simulink model "gm_HDLRx_vs"  (R2024a)
settings: Solver=FixedStepDiscrete  StartTime=0.0  StopTime=stopTime  RelTol=1e-3
undefined symbols (not defined in the file or in its folder): channelBitsPerSubcarrier, channelCyclicPrefixLen, channelOFDMSamples, channelScramblerInit, clk, clk_enable, decimatorDelay, decimatorFilter, fPHY, fs, headerBitsPerFec, headerBitsPerSubcarrier, headerCyclicPrefixLen, headerOFDMSamples, headerScramblerInit, lowerbound, N, numDataCarriers, payloadBitsPerFec, payloadScramblerInit, preambleBitsPerSubcarrier, preambleCyclicPrefixLen, preambleFirstPartOFDMSamples, preambleScramblerInit, preambleSecondPartOFDMSamples, QAM, reset_x, upperbound
libraries: hdlsllib x133, hdlmdlgenlib x132, simulink x8, whdlutilities x8, whdlmod x4, dspsrcs4 x2, whdledac x2, commhdlcrc x1, dsphdlfiltering2 x1, dsphdlsigops2 x1, vivadosimlib x1, HDL_ieee_8021513 x1
(part 2 of 4)

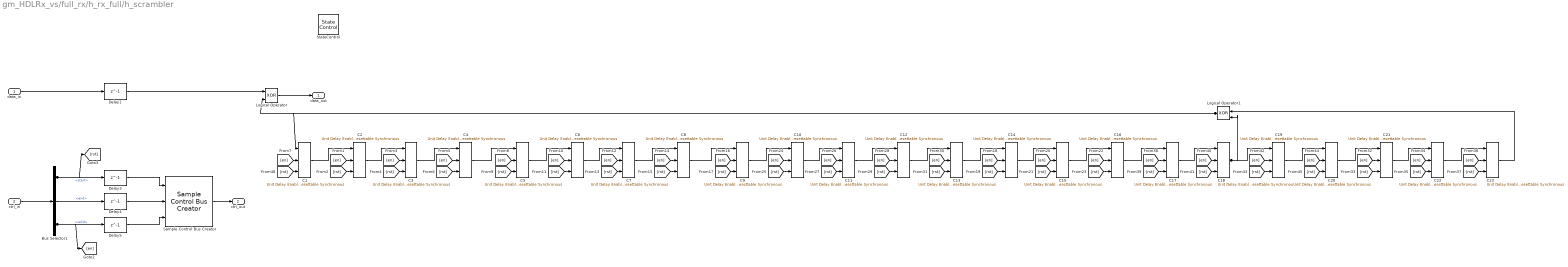
== system gm_HDLRx_vs/full_rx/h_rx_full/h_scrambler ==
  data_in : Inport  OutDataTypeStr=boolean  SampleTime=1e-08
  ctrl_in : Inport  Port=2  SampleTime=1e-08
  Bus Selector1 : BusSelector  OutputSignals=start,end,valid
  C{1,3,5,7,9,11,13,15,17,19,21,23} (12 alike) : hdlsllib/Discrete/Unit Delay Enabled Resettable Synchronous  InitialCondition=0  SampleTime=-1
  C{2,4,6,8,10,12,14,16,18,20,22} (11 alike) : hdlsllib/Discrete/Unit Delay Enabled Resettable Synchronous  InitialCondition=1  SampleTime=-1
  Delay{1,3..5} (4 alike) : Delay  DelayLength=1  InitialCondition=0  UseCircularBuffer=on
  Logical Operator : Logic  Operator=XOR  IconShape=distinctive  AllPortsSameDT=off  OutDataTypeStr=boolean
  Logical Operator1 : Logic  Operator=XOR  IconShape=distinctive  AllPortsSameDT=off  OutDataTypeStr=boolean
  Sample Control Bus Creator : whdlutilities/Sample Control Bus Creator
  StateControl : StateControl  StateControl=Synchronous
  data_out : Outport  SampleTime=1e-08
  ctrl_out : Outport  Port=2  SampleTime=1e-08
  wires:
  Sample Control Bus Creator/1 -> ctrl_out/1
  Logical Operator1/1 -> C1/1, Logical Operator/2
  Logical Operator/1 -> data_out/1
  [rst] -> C5/3
  [en] -> C5/2
  [en] -> C1/2
  [rst] -> C4/3
  [en] -> C4/2
  [rst] -> C1/3
  [rst] -> C20/3
  [en] -> C20/2
  [rst] -> C19/3
  [en] -> C19/2
  [rst] -> C18/3
  [en] -> C18/2
  [rst] -> C3/3
  [rst] -> C17/3
  [en] -> C17/2
  [rst] -> C23/3
  [en] -> C23/2
  [rst] -> C22/3
  [en] -> C22/2
  [rst] -> C21/3
  [en] -> C21/2
  [rst] -> C13/3
  [en] -> C13/2
  [en] -> C3/2
  [rst] -> C12/3
  [en] -> C12/2
  [rst] -> C11/3
  [en] -> C11/2
  [rst] -> C10/3
  [en] -> C10/2
  [rst] -> C16/3
  [en] -> C16/2
  [rst] -> C15/3
  [en] -> C15/2
  [rst] -> C2/3
  [rst] -> C14/3
  [en] -> C14/2
  [rst] -> C9/3
  [en] -> C9/2
  [rst] -> C8/3
  [en] -> C8/2
  [rst] -> C7/3
  [en] -> C7/2
  [rst] -> C6/3
  [en] -> C6/2
  [en] -> C2/2
  Delay5/1 -> Sample Control Bus Creator/3
  Delay4/1 -> Sample Control Bus Creator/2
  Delay3/1 -> Sample Control Bus Creator/1
  Delay1/1 -> Logical Operator/1
  C9/1 -> C10/1
  C8/1 -> C9/1
  C7/1 -> C8/1
  C6/1 -> C7/1
  C5/1 -> C6/1
  C4/1 -> C5/1
  C3/1 -> C4/1
  C23/1 -> Logical Operator1/1
  C22/1 -> C23/1
  C21/1 -> C22/1
  C20/1 -> C21/1
  C2/1 -> C3/1
  C19/1 -> C20/1
  C18/1 -> C19/1, Logical Operator1/2
  C17/1 -> C18/1
  C16/1 -> C17/1
  C15/1 -> C16/1
  C14/1 -> C15/1
  C13/1 -> C14/1
  C12/1 -> C13/1
  C11/1 -> C12/1
  C10/1 -> C11/1
  C1/1 -> C2/1
  Bus Selector1/3 -> Delay5/1, [en]  "<valid>"
  Bus Selector1/2 -> Delay4/1  "<end>"
  Bus Selector1/1 -> Delay3/1, [rst]  "<start>"
  ctrl_in/1 -> Bus Selector1/1
  data_in/1 -> Delay1/1

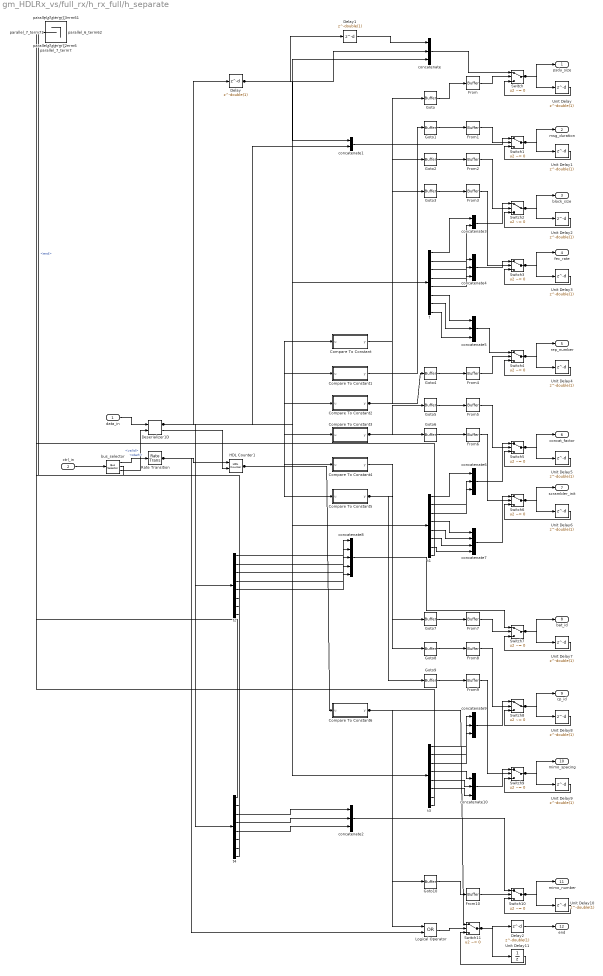
== system gm_HDLRx_vs/full_rx/h_rx_full/h_separate ==
  data_in : Inport  OutDataTypeStr=boolean  SampleTime=1e-08
  ctrl_in : Inport  Port=2  SampleTime=1e-08
  Compare To Constant : Subsystem  mask(Compare To Constant){relop===, const=double(3), OutDataTypeStr=boolean, ZeroCross=on}
      mask prompts: relop "Simulink:masks:Operator_MP"; const "Simulink:masks:ConstantValue_MP"; OutDataTypeStr "Simulink:masks:OutputDataType_MP"; ZeroCross "Simulink:masks:EnableZerocrossingDetection_MP"
      mask help: Simulink:masks:CompareToConstant_MD
      mask init:
      | OutDataTypeStr = 'boolean';
      | ZeroCross = 'on';
      | blkName = 'HDLRx/full_rx/h_rx_full/h_separate/Compare\nTo Constant';
      | const = double(3);
      | const_str = '3';
      | const_val = double(3);
      | relop = '==';
      | setValue = 'boolean';
      | str = '== 3';
      mask TypeOptions relop: == | ~= | < | <= | >= | >
      mask TypeOptions OutDataTypeStr: Simulink:masks:uint8 | Simulink:masks:boolean
      mask Callback ZeroCross: sl('zeroCrossEnable', gcbh);
      mask Display: disp(str)
  Compare To Constant1 : Subsystem  mask(Compare To Constant){relop===, const=double(5), OutDataTypeStr=boolean, ZeroCross=on}
      mask prompts: relop "Simulink:masks:Operator_MP"; const "Simulink:masks:ConstantValue_MP"; OutDataTypeStr "Simulink:masks:OutputDataType_MP"; ZeroCross "Simulink:masks:EnableZerocrossingDetection_MP"
      mask help: Simulink:masks:CompareToConstant_MD
      mask init:
      | OutDataTypeStr = 'boolean';
      | ZeroCross = 'on';
      | blkName = 'HDLRx/full_rx/h_rx_full/h_separate/Compare\nTo Constant1';
      | const = double(5);
      | const_str = '5';
      | const_val = double(5);
      | relop = '==';
      | setValue = 'boolean';
      | str = '== 5';
      mask TypeOptions relop: == | ~= | < | <= | >= | >
      mask TypeOptions OutDataTypeStr: Simulink:masks:uint8 | Simulink:masks:boolean
      mask Callback ZeroCross: sl('zeroCrossEnable', gcbh);
      mask Display: disp(str)
  Compare To Constant2 : Subsystem  mask(Compare To Constant){relop===, const=double(6), OutDataTypeStr=boolean, ZeroCross=on}
      mask prompts: relop "Simulink:masks:Operator_MP"; const "Simulink:masks:ConstantValue_MP"; OutDataTypeStr "Simulink:masks:OutputDataType_MP"; ZeroCross "Simulink:masks:EnableZerocrossingDetection_MP"
      mask help: Simulink:masks:CompareToConstant_MD
      mask init:
      | OutDataTypeStr = 'boolean';
      | ZeroCross = 'on';
      | blkName = 'HDLRx/full_rx/h_rx_full/h_separate/Compare\nTo Constant2';
      | const = double(6);
      | const_str = '6';
      | const_val = double(6);
      | relop = '==';
      | setValue = 'boolean';
      | str = '== 6';
      mask TypeOptions relop: == | ~= | < | <= | >= | >
      mask TypeOptions OutDataTypeStr: Simulink:masks:uint8 | Simulink:masks:boolean
      mask Callback ZeroCross: sl('zeroCrossEnable', gcbh);
      mask Display: disp(str)
  Compare To Constant3 : Subsystem  mask(Compare To Constant){relop===, const=double(7), OutDataTypeStr=boolean, ZeroCross=on}
      mask prompts: relop "Simulink:masks:Operator_MP"; const "Simulink:masks:ConstantValue_MP"; OutDataTypeStr "Simulink:masks:OutputDataType_MP"; ZeroCross "Simulink:masks:EnableZerocrossingDetection_MP"
      mask help: Simulink:masks:CompareToConstant_MD
      mask init:
      | OutDataTypeStr = 'boolean';
      | ZeroCross = 'on';
      | blkName = 'HDLRx/full_rx/h_rx_full/h_separate/Compare\nTo Constant3';
      | const = double(7);
      | const_str = '7';
      | const_val = double(7);
      | relop = '==';
      | setValue = 'boolean';
      | str = '== 7';
      mask TypeOptions relop: == | ~= | < | <= | >= | >
      mask TypeOptions OutDataTypeStr: Simulink:masks:uint8 | Simulink:masks:boolean
      mask Callback ZeroCross: sl('zeroCrossEnable', gcbh);
      mask Display: disp(str)
  Compare To Constant4 : Subsystem  mask(Compare To Constant){relop===, const=double(8), OutDataTypeStr=boolean, ZeroCross=on}
      mask prompts: relop "Simulink:masks:Operator_MP"; const "Simulink:masks:ConstantValue_MP"; OutDataTypeStr "Simulink:masks:OutputDataType_MP"; ZeroCross "Simulink:masks:EnableZerocrossingDetection_MP"
      mask help: Simulink:masks:CompareToConstant_MD
      mask init:
      | OutDataTypeStr = 'boolean';
      | ZeroCross = 'on';
      | blkName = 'HDLRx/full_rx/h_rx_full/h_separate/Compare\nTo Constant4';
      | const = double(8);
      | const_str = '8';
      | const_val = double(8);
      | relop = '==';
      | setValue = 'boolean';
      | str = '== 8';
      mask TypeOptions relop: == | ~= | < | <= | >= | >
      mask TypeOptions OutDataTypeStr: Simulink:masks:uint8 | Simulink:masks:boolean
      mask Callback ZeroCross: sl('zeroCrossEnable', gcbh);
      mask Display: disp(str)
  Compare To Constant5 : Subsystem  mask(Compare To Constant){relop===, const=double(9), OutDataTypeStr=boolean, ZeroCross=on}
      mask prompts: relop "Simulink:masks:Operator_MP"; const "Simulink:masks:ConstantValue_MP"; OutDataTypeStr "Simulink:masks:OutputDataType_MP"; ZeroCross "Simulink:masks:EnableZerocrossingDetection_MP"
      mask help: Simulink:masks:CompareToConstant_MD
      mask init:
      | OutDataTypeStr = 'boolean';
      | ZeroCross = 'on';
      | blkName = 'HDLRx/full_rx/h_rx_full/h_separate/Compare\nTo Constant5';
      | const = double(9);
      | const_str = '9';
      | const_val = double(9);
      | relop = '==';
      | setValue = 'boolean';
      | str = '== 9';
      mask TypeOptions relop: == | ~= | < | <= | >= | >
      mask TypeOptions OutDataTypeStr: Simulink:masks:uint8 | Simulink:masks:boolean
      mask Callback ZeroCross: sl('zeroCrossEnable', gcbh);
      mask Display: disp(str)
  Compare To Constant6 : Subsystem  mask(Compare To Constant){relop===, const=double(13), OutDataTypeStr=boolean, ZeroCross=on}
      mask prompts: relop "Simulink:masks:Operator_MP"; const "Simulink:masks:ConstantValue_MP"; OutDataTypeStr "Simulink:masks:OutputDataType_MP"; ZeroCross "Simulink:masks:EnableZerocrossingDetection_MP"
      mask help: Simulink:masks:CompareToConstant_MD
      mask init:
      | OutDataTypeStr = 'boolean';
      | ZeroCross = 'on';
      | blkName = 'HDLRx/full_rx/h_rx_full/h_separate/Compare\nTo Constant6';
      | const = double(13);
      | const_str = '13';
      | const_val = double(13);
      | relop = '==';
      | setValue = 'boolean';
      | str = '== 13';
      mask TypeOptions relop: == | ~= | < | <= | >= | >
      mask TypeOptions OutDataTypeStr: Simulink:masks:uint8 | Simulink:masks:boolean
      mask Callback ZeroCross: sl('zeroCrossEnable', gcbh);
      mask Display: disp(str)
  Delay : Delay  DelayLength=double(1)  InitialCondition=0  SampleTime=8e-08
  Delay1 : Delay  DelayLength=double(1)  InitialCondition=0  SampleTime=8e-08
  Delay2 : Delay  DelayLength=double(1)  InitialCondition=0  SampleTime=8e-08
  Deserializer1D : hdlsllib/HDL Operations/Deserializer1D  Ratio=8  IdleCycles=0  InitialCondition=0  startIn=off  validIn=on  validOut=on  inputDataDimensions=1  inputSampleTime=1e-08  inputSignalType=real
  From{,1..10} (11 alike) : hdlmdlgenlib/Buffer
  Goto{,1..10} (11 alike) : hdlmdlgenlib/Buffer
  HDL Counter1 : hdlsllib/Sources/HDL Counter  CountType=Free running  CountInit=0  CountStep=1  CountMax=25  CountFromType=Initial value  CountFrom=0  CountResetPort=on  CountLoadPort=off  CountEnbPort=on  CountDirPort=off  CountHitOutputPort=off  CountDataType=Unsigned  CountWordLen=5  CountFracLen=0  CountSampTime=1
  Logical Operator : Logic  Operator=OR  AllPortsSameDT=off  OutDataTypeStr=boolean  SampleTime=8e-08
  Rate Transition : RateTransition  InitialCondition=double(0)  OutPortSampleTimeOpt=Multiple of input port sample time  OutPortSampleTimeMultiple=8
  Switch{,1..10} (11 alike) : Switch  Criteria=u2 ~= 0  Threshold=double(0)  OutDataTypeStr=fixdt(0, 1, 0)  SampleTime=8e-08  SaturateOnIntegerOverflow=off  InputSameDT=off
  Switch11 : Switch  Criteria=u2 ~= 0  Threshold=double(0)  OutDataTypeStr=boolean  SampleTime=8e-08  SaturateOnIntegerOverflow=off  InputSameDT=off
  Unit Delay{,1..10} (11 alike) : Delay  DelayLength=double(1)  InitialCondition=0  SampleTime=8e-08
  Unit Delay11 : UnitDelay  SampleTime=8e-08
  bus_selector : BusSelector  OutputSignals=start,end,valid
  bus_selector_term1 : Terminator
  concatenate{,2,4..6,9..10} (7 alike) : Concatenate  NumInputs=3
  concatenate1 : Concatenate
  concatenate3 : Concatenate
  concatenate7 : Concatenate  NumInputs=4
  concatenate8 : Concatenate  NumInputs=5
  parallel_0_term0 : Terminator
  parallel_1_term1 : Terminator
  parallel_5_term5 : Terminator
  parallel_5_term51 : Terminator
  parallel_6_term6 : Terminator
  parallel_6_term61 : Terminator
  parallel_6_term62 : Terminator
  parallel_7_term{7,71..73} (4 alike) : Terminator
  t{,1..4} (5 alike) : Demux  Outputs=8
  psdu_size : Outport  SampleTime=8e-08
  msg_duration : Outport  Port=2  SampleTime=8e-08
  block_size : Outport  Port=3  SampleTime=8e-08
  fec_rate : Outport  Port=4  SampleTime=8e-08
  rep_number : Outport  Port=5  SampleTime=8e-08
  concat_factor : Outport  Port=6  SampleTime=8e-08
  scrambler_init : Outport  Port=7  SampleTime=8e-08
  bat_id : Outport  Port=8  SampleTime=8e-08
  cp_id : Outport  Port=9  SampleTime=8e-08
  mimo_spacing : Outport  Port=10  SampleTime=8e-08
  mimo_number : Outport  Port=11  SampleTime=8e-08
  end : Outport  Port=12  SampleTime=8e-08
  wires:
  t4/8 -> parallel_7_term7/1
  t4/7 -> parallel_6_term61/1
  t4/6 -> parallel_5_term5/1
  t4/5 -> concatenate2/3
  t4/4 -> concatenate2/2
  t4/3 -> concatenate2/1
  t4/2 -> parallel_1_term1/1
  t4/1 -> parallel_0_term0/1
  t3/8 -> parallel_7_term71/1
  t3/7 -> parallel_6_term62/1
  t3/6 -> concatenate10/3
  t3/5 -> concatenate10/2
  t3/4 -> concatenate10/1
  t3/3 -> concatenate9/3
  t3/2 -> concatenate9/2
  t3/1 -> concatenate9/1
  t2/8 -> parallel_7_term72/1
  t2/7 -> parallel_6_term6/1
  t2/6 -> parallel_5_term51/1
  t2/5 -> concatenate8/5
  t2/4 -> concatenate8/4
  t2/3 -> concatenate8/3
  t2/2 -> concatenate8/2
  t2/1 -> concatenate8/1
  t1/8 -> parallel_7_term73/1
  t1/7 -> concatenate7/4
  t1/6 -> concatenate7/3
  t1/5 -> concatenate7/2
  t1/4 -> concatenate7/1
  t1/3 -> concatenate6/3
  t1/2 -> concatenate6/2
  t1/1 -> concatenate6/1
  t/8 -> concatenate5/3
  t/7 -> concatenate5/2
  t/6 -> concatenate5/1
  t/5 -> concatenate4/3
  t/4 -> concatenate4/2
  t/3 -> concatenate4/1
  t/2 -> concatenate3/2
  t/1 -> concatenate3/1
  Goto9/1 -> From9/1
  Goto8/1 -> From8/1
  Goto7/1 -> From7/1
  Goto6/1 -> From6/1
  Goto5/1 -> From5/1
  Goto4/1 -> From4/1
  Goto3/1 -> From3/1
  Goto2/1 -> From2/1
  Goto10/1 -> From10/1
  Goto1/1 -> From1/1
  Goto/1 -> From/1
  concatenate10/1 -> Switch9/1
  concatenate9/1 -> Switch8/1
  concatenate8/1 -> Switch7/1
  concatenate7/1 -> Switch6/1
  concatenate6/1 -> Switch5/1
  concatenate5/1 -> Switch4/1
  concatenate4/1 -> Switch3/1
  concatenate3/1 -> Switch2/1
  concatenate2/1 -> Switch10/1
  concatenate1/1 -> Switch1/1
  concatenate/1 -> Switch/1
  Unit Delay9/1 -> Switch9/3
  Unit Delay8/1 -> Switch8/3
  Unit Delay7/1 -> Switch7/3
  Unit Delay6/1 -> Switch6/3
  Unit Delay5/1 -> Switch5/3
  Unit Delay4/1 -> Switch4/3
  Unit Delay3/1 -> Switch3/3
  Unit Delay2/1 -> Switch2/3
  Unit Delay11/1 -> Switch11/3
  Unit Delay10/1 -> Switch10/3
  Unit Delay1/1 -> Switch1/3
  Unit Delay/1 -> Switch/3
  Switch9/1 -> mimo_spacing/1, Unit Delay9/1
  Switch8/1 -> cp_id/1, Unit Delay8/1
  Switch7/1 -> bat_id/1, Unit Delay7/1
  Switch6/1 -> scrambler_init/1, Unit Delay6/1
  Switch5/1 -> concat_factor/1, Unit Delay5/1
  Switch4/1 -> rep_number/1, Unit Delay4/1
  Switch3/1 -> fec_rate/1, Unit Delay3/1
  Switch2/1 -> block_size/1, Unit Delay2/1
  Switch11/1 -> Delay2/1, Unit Delay11/1
  Switch10/1 -> mimo_number/1, Unit Delay10/1
  Switch1/1 -> msg_duration/1, Unit Delay1/1
  Switch/1 -> psdu_size/1, Unit Delay/1
  bus_selector/3 -> Deserializer1D/2  "<valid>"
  bus_selector/2 -> bus_selector_term1/1  "<end>"
  bus_selector/1 -> Rate Transition/1  "<start>"
  Rate Transition/1 -> HDL Counter1/1, Logical Operator/2
  Logical Operator/1 -> Switch11/2
  HDL Counter1/1 -> Compare To Constant/1(u), Compare To Constant1/1(u), Compare To Constant2/1(u), Compare To Constant3/1(u), Compare To Constant4/1(u), Compare To Constant5/1(u), Compare To Constant6/1(u)
  From9/1 -> Switch9/2
  From8/1 -> Switch8/2
  From7/1 -> Switch7/2
  From6/1 -> Switch6/2
  From5/1 -> Switch5/2
  From4/1 -> Switch4/2
  From3/1 -> Switch3/2
  From2/1 -> Switch2/2
  From10/1 -> Switch10/2
  From1/1 -> Switch1/2
  From/1 -> Switch/2
  Deserializer1D/2 -> HDL Counter1/2
  Deserializer1D/1 -> Delay/1, t/1, t1/1, t2/1, t3/1, t4/1, concatenate/3, concatenate1/2
  Delay2/1 -> end/1
  Delay1/1 -> concatenate/1
  Delay/1 -> Delay1/1, concatenate/2, concatenate1/1
  Compare To Constant6/1(y) -> Goto10/1, Logical Operator/1, Switch11/1
  Compare To Constant5/1(y) -> Goto8/1, Goto9/1
  Compare To Constant4/1(y) -> Goto7/1
  Compare To Constant3/1(y) -> Goto5/1, Goto6/1
  Compare To Constant2/1(y) -> Goto2/1, Goto3/1, Goto4/1
  Compare To Constant1/1(y) -> Goto1/1
  Compare To Constant/1(y) -> Goto/1
  ctrl_in/1 -> bus_selector/1
  data_in/1 -> Deserializer1D/1

== system gm_HDLRx_vs/full_rx/header_clock_x2/rising_edge_detector ==
  In : Inport  OutDataTypeStr=boolean  SampleTime=1e-08
  Delay2 : Delay  DelayLength=1  InitialCondition=0  UseCircularBuffer=on
  Logical Operator1 : Logic  IconShape=distinctive  AllPortsSameDT=off  OutDataTypeStr=boolean
  Logical Operator2 : Logic  Operator=NOT  IconShape=distinctive  AllPortsSameDT=off  OutDataTypeStr=boolean
  Out : Outport  SampleTime=1e-08
  wires:
  Logical Operator2/1 -> Logical Operator1/2
  Logical Operator1/1 -> Out/1
  Delay2/1 -> Logical Operator2/1
  In/1 -> Delay2/1, Logical Operator1/1

== system gm_HDLRx_vs/full_rx/prepare_payload_data/falling_edge_detector ==
  in : Inport  OutDataTypeStr=boolean  SampleTime=1e-08
  Delay : Delay  DelayLength=1  InitialCondition=0  UseCircularBuffer=on
  Logical Operator : Logic  IconShape=distinctive  AllPortsSameDT=off  OutDataTypeStr=boolean
  Logical Operator1 : Logic  Operator=NOT  IconShape=distinctive  AllPortsSameDT=off  OutDataTypeStr=boolean
  out : Outport  SampleTime=1e-08
  wires:
  Logical Operator1/1 -> Logical Operator/1
  Logical Operator/1 -> out/1
  Delay/1 -> Logical Operator/2
  in/1 -> Delay/1, Logical Operator1/1

== system gm_HDLRx_vs/full_rx/prepare_payload_data/payload_clock_x2 ==
  data_in : Inport  OutDataTypeStr=fixdt(1, 16, 12)  PortDimensions=[4 1]  SampleTime=2e-08
  valid_in : Inport  Port=2  OutDataTypeStr=boolean  PortDimensions=1  SampleTime=2e-08
  Serializer1D : hdlsllib/HDL Operations/Serializer1D  Ratio=2  IdleCycles=0  validIn=on  startOut=off  validOut=on  inputDataDimensions=2  inputSampleTime=2e-08  inputSignalType=real
  concatenate : Concatenate  Mode=Multidimensional array
  data_in_0_term0 : Terminator
  data_in_1_term1 : Terminator
  t : Demux
  data_out : Outport  SampleTime=1e-08
  valid_out : Outport  Port=2  SampleTime=1e-08
  wires:
  t/4 -> concatenate/2
  t/3 -> concatenate/1
  t/2 -> data_in_1_term1/1
  t/1 -> data_in_0_term0/1
  concatenate/1 -> Serializer1D/1
  Serializer1D/2 -> valid_out/1
  Serializer1D/1 -> data_out/1
  valid_in/1 -> Serializer1D/2
  data_in/1 -> t/1

== system gm_HDLRx_vs/full_rx/prepare_payload_data/rising_edge_detector ==
  In : Inport  OutDataTypeStr=boolean  SampleTime=1e-08
  Delay2 : Delay  DelayLength=1  InitialCondition=0  UseCircularBuffer=on
  Logical Operator1 : Logic  IconShape=distinctive  AllPortsSameDT=off  OutDataTypeStr=boolean
  Logical Operator2 : Logic  Operator=NOT  IconShape=distinctive  AllPortsSameDT=off  OutDataTypeStr=boolean
  Out : Outport  SampleTime=1e-08
  wires:
  Logical Operator2/1 -> Logical Operator1/2
  Logical Operator1/1 -> Out/1
  Delay2/1 -> Logical Operator2/1
  In/1 -> Delay2/1, Logical Operator1/1

== system gm_HDLRx_vs/full_rx/rx_demodulator_full/constellation_descrambler ==
  data_in : Inport  OutDataTypeStr=fixdt(1, 24, 12)  SampleTime=2e-08
      settings: SignalType=complex
  valid_in : Inport  Port=2  OutDataTypeStr=boolean  SampleTime=2e-08
  init : Inport  Port=3  OutDataTypeStr=boolean  PortDimensions=[13]  SampleTime=2e-08
  rising_edge_detector : Subsystem
  rotate_-90 : Subsystem
  sync_constellation_scrambler : Subsystem
  data_out : Outport  SampleTime=2e-08
  valid_out : Outport  Port=2  SampleTime=2e-08
  wires:
  sync_constellation_scrambler/2(s2) -> rotate_-90/4(s2_in)
  sync_constellation_scrambler/1(s1) -> rotate_-90/3(s1_in)
  rotate_-90/2(valid_out) -> valid_out/1
  rotate_-90/1(data_out) -> data_out/1
  rising_edge_detector/1(Out) -> sync_constellation_scrambler/1(new_ofdm_symbol)
  init/1 -> sync_constellation_scrambler/2(init)
  valid_in/1 -> sync_constellation_scrambler/3(valid_in), rotate_-90/2(valid_in), rising_edge_detector/1(In)
  data_in/1 -> rotate_-90/1(data_in)

== system gm_HDLRx_vs/full_rx/rx_demodulator_full/decimator ==
  data_in : Inport  OutDataTypeStr=fixdt(1, 16, 12)  SampleTime=1e-08
      settings: SignalType=complex
  valid_in : Inport  Port=2  OutDataTypeStr=boolean  SampleTime=1e-08
  Delay : Delay  InitialCondition=0  UseCircularBuffer=on
  Delay1 : Delay  DelayLength=decimatorDelay/2  InitialCondition=0  UseCircularBuffer=on
  Delay2 : Delay  InitialCondition=0  UseCircularBuffer=on
  Delay3 : Delay  DelayLength=(decimatorDelay-2)*4  InitialCondition=0  UseCircularBuffer=on
  Delay4 : Delay  DelayLength=1  InitialCondition=0  UseCircularBuffer=on
  Delay5 : Delay  DelayLength=1  InitialCondition=0  UseCircularBuffer=on
  FIR Decimator : dsphdlfiltering2/FIR Decimator  Numerator=decimatorFilter.Numerator  FilterStructure=Direct form systolic  DecimationFactor=oversamplingFactor  NumCycles=1  SimulateUsing=Code generation  roundingMode=Floor  overflowMode=off  CoefficientsDataTypeStr=fixdt(1,16)  OutputDataTypeStr=fixdt(1,16,12)  ResetInputPort=on  HDLGlobalReset=off
  Logical Operator : Logic  Operator=OR  IconShape=distinctive  AllPortsSameDT=off  OutDataTypeStr=boolean
  Logical Operator1 : Logic  IconShape=distinctive  AllPortsSameDT=off  OutDataTypeStr=boolean
  Rate Transition : RateTransition  OutPortSampleTimeOpt=Multiple of input port sample time  OutPortSampleTimeMultiple=oversamplingFactor
  Rate Transition1 : RateTransition  OutPortSampleTimeOpt=Multiple of input port sample time  OutPortSampleTimeMultiple=oversamplingFactor
  rising_edge_detector : Subsystem
  data_out : Outport  SampleTime=2e-08
  valid_out : Outport  Port=2  SampleTime=2e-08
  wires:
  rising_edge_detector/1(Out) -> FIR Decimator/3
  Rate Transition1/1 -> data_out/1
  Rate Transition/1 -> Delay1/1, Logical Operator1/1
  Logical Operator1/1 -> valid_out/1
  Logical Operator/1 -> FIR Decimator/2
  FIR Decimator/2 -> Rate Transition/1
  FIR Decimator/1 -> Rate Transition1/1
  Delay5/1 -> rising_edge_detector/1(In)
  Delay4/1 -> FIR Decimator/1
  Delay3/1 -> Logical Operator/2
  Delay2/1 -> Delay4/1
  Delay1/1 -> Logical Operator1/2
  Delay/1 -> Delay3/1, Logical Operator/1
  valid_in/1 -> Delay/1, Delay5/1
  data_in/1 -> Delay2/1

== system gm_HDLRx_vs/full_rx/rx_demodulator_full/downshifter ==
  data_in : Inport  OutDataTypeStr=fixdt(1, 16, 12)  SampleTime=1e-08
  valid_in : Inport  Port=2  OutDataTypeStr=boolean  SampleTime=1e-08
  Delay : Delay  DelayLength=6  InitialCondition=0  UseCircularBuffer=on
  Delay1 : Delay  DelayLength=4  InitialCondition=0  UseCircularBuffer=on
  Delay2 : Delay  DelayLength=1  InitialCondition=0  UseCircularBuffer=on
  Delay3 : Delay  DelayLength=1  InitialCondition=0  UseCircularBuffer=on
  NCO : dsphdlsigops2/NCO  PhaseIncrementSource=Property  PhaseIncrement=ncoPhaseIncrement  PhaseOffsetSource=Property  PhaseOffset=0  DitherSource=None  NumDitherBits=1  SamplesPerFrame=1  LUTCompress=off  ResetAction=on  Waveform=Complex exponential  PhasePort=off  SimulateUsing=Code generation  AccumulatorWL=ncoWordLength  PhaseQuantization=off  NumQuantizerAccumulatorBits=6  OutputDataType=Binary point scaling  OutputWL=16  OutputFL=12
  digital_carrier_receiver : Subsystem
  rising_edge_detector : Subsystem
  data_out : Outport  SampleTime=1e-08
  valid_out : Outport  Port=2  SampleTime=1e-08
  wires:
  rising_edge_detector/1(Out) -> NCO/1
  digital_carrier_receiver/1(data_out) -> data_out/1
  NCO/2 -> Delay1/1
  NCO/1 -> digital_carrier_receiver/2(ncoIn)
  Delay3/1 -> Delay/1
  Delay2/1 -> NCO/2
  Delay1/1 -> valid_out/1
  Delay/1 -> digital_carrier_receiver/1(dataIn)
  valid_in/1 -> rising_edge_detector/1(In), Delay2/1
  data_in/1 -> Delay3/1

== system gm_HDLRx_vs/full_rx/rx_demodulator_full/ofdm_demod ==
  data_in : Inport  OutDataTypeStr=fixdt(1, 16, 12)  SampleTime=2e-08
      settings: SignalType=complex
  valid_in : Inport  Port=2  OutDataTypeStr=boolean  SampleTime=2e-08
  cp_len : Inport  Port=3  OutDataTypeStr=uint8  SampleTime=2e-08
  Constant2 : Constant  Value=N  OutDataTypeStr=fixdt(0,9,0)  SampleTime=-1  LockScale=on
  Constant3 : Constant  Value=0  OutDataTypeStr=fixdt(0,2,0)  SampleTime=-1  LockScale=on
  Constant4 : Constant  Value=11  OutDataTypeStr=fixdt(0,4,0)  SampleTime=-1  LockScale=on
  OFDM Demodulator : whdlmod/OFDM Demodulator  OFDMParamsSource=Input port  MaxFFTLength=N  FFTLength=64  CPLength=16  NumLGsC=6  NumRGsC=5  CPFraction=off  CPFractionSource=Property  CPFractionValue=0.55  removeDCSubcarriers=off  enableResetInputPort=off  Normalize=off  RoundingMethod=Floor  SimulateUsing=Code generation
  data_out : Outport  SampleTime=2e-08
  valid_out : Outport  Port=2  SampleTime=2e-08
  ready : Outport  Port=3  SampleTime=2e-08
  wires:
  OFDM Demodulator/3 -> ready/1
  OFDM Demodulator/2 -> valid_out/1
  OFDM Demodulator/1 -> data_out/1
  Constant4/1 -> OFDM Demodulator/5
  Constant3/1 -> OFDM Demodulator/6
  Constant2/1 -> OFDM Demodulator/3
  cp_len/1 -> OFDM Demodulator/4
  valid_in/1 -> OFDM Demodulator/2
  data_in/1 -> OFDM Demodulator/1

== system gm_HDLRx_vs/full_rx/rx_demodulator_full/ofdm_rx_counter ==
  note: Counts the amount of OFDM symbols for every "end" signal, and assigns them a position (preamble, channel, header, payload)
  valid : Inport  OutDataTypeStr=boolean  PortDimensions=1  SampleTime=2e-08
  rst : Inport  Port=2  OutDataTypeStr=boolean  PortDimensions=1  SampleTime=2e-08
  payload_num_ofdm_symbols : Inport  Port=3  OutDataTypeStr=fixdt(1, 17, 0)  PortDimensions=1  SampleTime=2e-08
  Add : Sum  OutDataTypeStr=fixdt(1, 18, 0)
  Constant : Constant  Value=3  OutDataTypeStr=uint16  SampleTime=-1
  Constant1 : Constant  Value=5  OutDataTypeStr=uint16  SampleTime=-1
  Constant2 : Constant  Value=6  OutDataTypeStr=uint16  SampleTime=-1
  Constant3 : Constant  Value=6  OutDataTypeStr=uint16  SampleTime=-1
  HDL Counter : hdlsllib/Sources/HDL Counter  CountType=Free running  CountInit=0  CountStep=1  CountMax=25  CountFromType=Initial value  CountFrom=0  CountResetPort=on  CountLoadPort=off  CountEnbPort=on  CountDirPort=off  CountHitOutputPort=off  CountDataType=Unsigned  CountWordLen=16  CountFracLen=0  CountSampTime=1
  Logical Operator : Logic  IconShape=distinctive  AllPortsSameDT=off  OutDataTypeStr=boolean
  Logical Operator1 : Logic  Operator=NOT  IconShape=distinctive  AllPortsSameDT=off  OutDataTypeStr=boolean
  Logical Operator2 : Logic  IconShape=distinctive  AllPortsSameDT=off  OutDataTypeStr=boolean
  Logical Operator3 : Logic  Operator=NOT  IconShape=distinctive  AllPortsSameDT=off  OutDataTypeStr=boolean
  Logical Operator4 : Logic  Operator=NOT  IconShape=distinctive  AllPortsSameDT=off  OutDataTypeStr=boolean
  Logical Operator5 : Logic  IconShape=distinctive  AllPortsSameDT=off  OutDataTypeStr=boolean
  Relational Operator{,1..3} (4 alike) : RelationalOperator  Operator=<=  OutDataTypeStr=boolean  InputSameDT=off
  falling_edge_detector1 : Subsystem
  rising_edge_detector1 : Subsystem
  is_channel : Outport  SampleTime=2e-08
  is_header : Outport  Port=2  SampleTime=2e-08
  is_payload : Outport  Port=3  SampleTime=2e-08
  wires:
  rising_edge_detector1/1(Out) -> HDL Counter/1
  falling_edge_detector1/1(out) -> HDL Counter/2
  Relational Operator3/1 -> Logical Operator5/2
  Relational Operator2/1 -> Logical Operator2/2, Logical Operator4/1
  Relational Operator1/1 -> Logical Operator/2, Logical Operator3/1
  Relational Operator/1 -> Logical Operator1/1
  Logical Operator5/1 -> is_payload/1
  Logical Operator4/1 -> Logical Operator5/1
  Logical Operator3/1 -> Logical Operator2/1
  Logical Operator2/1 -> is_header/1
  Logical Operator1/1 -> Logical Operator/1
  Logical Operator/1 -> is_channel/1
  HDL Counter/1 -> Relational Operator/1, Relational Operator1/1, Relational Operator2/1, Relational Operator3/1
  Constant3/1 -> Add/1
  Constant2/1 -> Relational Operator2/2
  Constant1/1 -> Relational Operator1/2
  Constant/1 -> Relational Operator/2
  Add/1 -> Relational Operator3/2
  payload_num_ofdm_symbols/1 -> Add/2
  rst/1 -> rising_edge_detector1/1(In)
  valid/1 -> falling_edge_detector1/1(in)

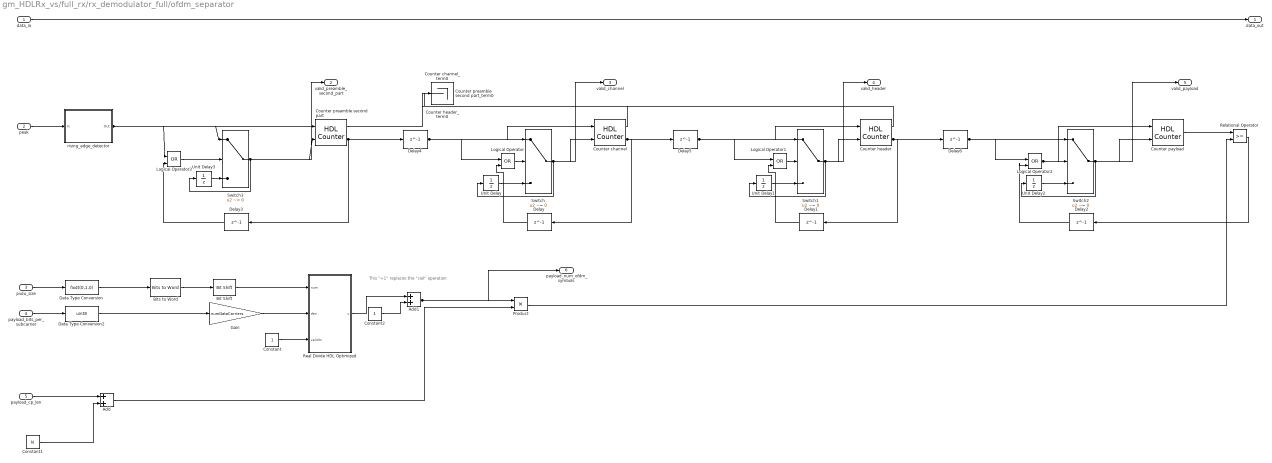
== system gm_HDLRx_vs/full_rx/rx_demodulator_full/ofdm_separator ==
  note: This "+1" replaces the "ceil" operation
  data_in : Inport  OutDataTypeStr=fixdt(1, 16, 12)  SampleTime=2e-08
      settings: SignalType=complex
  peak : Inport  Port=2  OutDataTypeStr=boolean  SampleTime=2e-08
  psdu_size : Inport  Port=3  OutDataTypeStr=fixdt(0, 1, 0)  PortDimensions=[24]  SampleTime=2e-08
  payload_bits_per_subcarrier : Inport  Port=4  OutDataTypeStr=fixdt(0, 4, 0)  SampleTime=2e-08
  payload_cp_len : Inport  Port=5  OutDataTypeStr=uint8  SampleTime=2e-08
  Add : Sum  OutDataTypeStr=fixdt(0, 10, 0)
  Add1 : Sum  OutDataTypeStr=fixdt(1, 17, 0)
  Bit Shift : hdlsllib/Logic and Bit Operations/Bit Shift  mode=Shift Left Logical  N=4
  Bits to Word : hdlsllib/Logic and Bit Operations/Bits to Word
  Constant : Constant  OutDataTypeStr=boolean  SampleTime=-1
  Constant1 : Constant  Value=N  OutDataTypeStr=fixdt(0,9,0)  SampleTime=-1
  Constant2 : Constant  OutDataTypeStr=fixdt(0,1,0)  SampleTime=-1
  Counter channel : hdlsllib/Sources/HDL Counter  CountType=Count limited  CountInit=0  CountStep=1  CountMax=channelOFDMSamples-2  CountFromType=Initial value  CountFrom=0  CountResetPort=on  CountLoadPort=off  CountEnbPort=on  CountDirPort=off  CountHitOutputPort=on  CountDataType=Unsigned  CountWordLen=nextpow2(channelOFDMSamples)  CountFracLen=0  CountSampTime=1
  Counter channel_term0 : Terminator
  Counter header : hdlsllib/Sources/HDL Counter  CountType=Count limited  CountInit=0  CountStep=1  CountMax=headerOFDMSamples-2  CountFromType=Initial value  CountFrom=0  CountResetPort=on  CountLoadPort=off  CountEnbPort=on  CountDirPort=off  CountHitOutputPort=on  CountDataType=Unsigned  CountWordLen=nextpow2(headerOFDMSamples)  CountFracLen=0  CountSampTime=1
  Counter header_term0 : Terminator
  Counter payload : hdlsllib/Sources/HDL Counter  CountType=Free running  CountInit=2  CountStep=1  CountMax=headerOFDMSamples-1  CountFromType=Initial value  CountFrom=2  CountResetPort=on  CountLoadPort=off  CountEnbPort=on  CountDirPort=off  CountHitOutputPort=off  CountDataType=Unsigned  CountWordLen=32  CountFracLen=0  CountSampTime=1
  Counter preamble second part : hdlsllib/Sources/HDL Counter  CountType=Count limited  CountInit=0  CountStep=1  CountMax=preambleSecondPartOFDMSamples-2  CountFromType=Initial value  CountFrom=0  CountResetPort=on  CountLoadPort=off  CountEnbPort=on  CountDirPort=off  CountHitOutputPort=on  CountDataType=Unsigned  CountWordLen=nextpow2(preambleSecondPartOFDMSamples)  CountFracLen=0  CountSampTime=1
  Counter preamble second part_term0 : Terminator
  Data Type Conversion : DataTypeConversion  OutDataTypeStr=fixdt(0,1,0)  SaturateOnIntegerOverflow=off  RndMeth=Floor
  Data Type Conversion2 : DataTypeConversion  OutDataTypeStr=uint8  SaturateOnIntegerOverflow=off  RndMeth=Floor
  Delay{,1..6} (7 alike) : Delay  DelayLength=1  InitialCondition=0  UseCircularBuffer=on
  Gain : Gain  Gain=numDataCarriers  OutDataTypeStr=uint16
  Logical Operator{,1..3} (4 alike) : Logic  Operator=OR  IconShape=distinctive  AllPortsSameDT=off  OutDataTypeStr=boolean
  Product : Product  OutDataTypeStr=fixdt(1, 27, 0)
  Real Divide HDL Optimized : Subsystem  mask(Real Divide HDL Optimized){OutputType=fixdt(1,16,0)}
      mask prompts: OutputType "fixed:emblib:OutputPrototype"
      mask help: fixed:emblib:RealDivideFullDescription
      mask Help: eval('embblk.embhelp(gcb)')
      mask Display:
      | text(0.5,0.6,'den ~= 0','texmode','on','HorizontalAlignment','center')
      | text(0.5,0.4,'y = num/den','texmode','on','HorizontalAlignment','center')
  Relational Operator : RelationalOperator  OutDataTypeStr=boolean  InputSameDT=off
  Switch{,1..3} (4 alike) : Switch  Criteria=u2 ~= 0  OutDataTypeStr=boolean  SaturateOnIntegerOverflow=off  InputSameDT=off
  Unit Delay{,1..3} (4 alike) : UnitDelay  SampleTime=-1  HasFrameUpgradeWarning=on
  rising_edge_detector : Subsystem
  data_out : Outport  SampleTime=2e-08
  valid_preamble_second_part : Outport  Port=2  SampleTime=2e-08
  valid_channel : Outport  Port=3  SampleTime=2e-08
  valid_header : Outport  Port=4  SampleTime=2e-08
  valid_payload : Outport  Port=5  SampleTime=2e-08
  payload_num_ofdm_symbols : Outport  Port=6  SampleTime=2e-08
  wires:
  rising_edge_detector/1(Out) -> Counter preamble second part/1, Logical Operator3/1, Switch3/1
  Unit Delay3/1 -> Switch3/3
  Unit Delay2/1 -> Switch2/3
  Unit Delay1/1 -> Switch1/3
  Unit Delay/1 -> Switch/3
  Switch3/1 -> Counter preamble second part/2, valid_preamble_second_part/1, Unit Delay3/1
  Switch2/1 -> Counter payload/2, valid_payload/1, Unit Delay2/1
  Switch1/1 -> Counter header/2, valid_header/1, Unit Delay1/1
  Switch/1 -> Counter channel/2, valid_channel/1, Unit Delay/1
  Relational Operator/1 -> Delay2/1
  Real Divide HDL Optimized/1(y) -> Add1/1
  Product/1 -> Relational Operator/2
  Logical Operator3/1 -> Switch3/2
  Logical Operator2/1 -> Counter payload/1, Switch2/2
  Logical Operator1/1 -> Switch1/2
  Logical Operator/1 -> Switch/2
  Gain/1 -> Real Divide HDL Optimized/2(den)
  Delay6/1 -> Logical Operator2/1, Switch2/1
  Delay5/1 -> Counter header/1, Logical Operator1/1, Switch1/1
  Delay4/1 -> Counter channel/1, Logical Operator/1, Switch/1
  Delay3/1 -> Logical Operator3/2
  Delay2/1 -> Logical Operator2/2
  Delay1/1 -> Logical Operator1/2
  Delay/1 -> Logical Operator/2
  Data Type Conversion2/1 -> Gain/1
  Data Type Conversion/1 -> Bits to Word/1
  Counter preamble second part/2 -> Delay3/1, Delay4/1
  Counter preamble second part/1 -> Counter preamble second part_term0/1
  Counter payload/1 -> Relational Operator/1
  Counter header/2 -> Delay1/1, Delay6/1
  Counter header/1 -> Counter header_term0/1
  Counter channel/2 -> Delay/1, Delay5/1
  Counter channel/1 -> Counter channel_term0/1
  Constant2/1 -> Add1/2
  Constant1/1 -> Add/2
  Constant/1 -> Real Divide HDL Optimized/3(validIn)
  Bits to Word/1 -> Bit Shift/1
  Bit Shift/1 -> Real Divide HDL Optimized/1(num)
  Add1/1 -> payload_num_ofdm_symbols/1, Product/1
  Add/1 -> Product/2
  payload_cp_len/1 -> Add/1
  payload_bits_per_subcarrier/1 -> Data Type Conversion2/1
  psdu_size/1 -> Data Type Conversion/1
  peak/1 -> rising_edge_detector/1(In)
  data_in/1 -> data_out/1

== system gm_HDLRx_vs/full_rx/rx_demodulator_full/qam_demod ==
  data_in : Inport  OutDataTypeStr=fixdt(1, 24, 12)  SampleTime=2e-08
      settings: SignalType=complex
  valid_in : Inport  Port=2  OutDataTypeStr=boolean  SampleTime=2e-08
  bits_per_subcarrier : Inport  Port=3  OutDataTypeStr=fixdt(0, 4, 0)  SampleTime=2e-08
  Constant{1..2,4..5} (4 alike) : Constant  Value=[0; 0; 0; 0]  VectorParams1D=off  OutDataTypeStr=fixdt(1, 28, 12)  SampleTime=-1  LockScale=on
  Delay : Delay  DelayLength=1  InitialCondition=0  UseCircularBuffer=on
  Delay1 : Delay  DelayLength=1  InitialCondition=0  UseCircularBuffer=on
  Delay2 : Delay  DelayLength=0  InitialCondition=0  UseCircularBuffer=on
  Delay3 : Delay  DelayLength=1  InitialCondition=0  UseCircularBuffer=on
  Delay4 : Delay  DelayLength=0  InitialCondition=0  UseCircularBuffer=on
  Delay5 : Delay  DelayLength=6  InitialCondition=0  UseCircularBuffer=on
  Delay7 : Delay  DelayLength=6  InitialCondition=0  UseCircularBuffer=on
  Multiport Switch : MultiPortSwitch  DataPortOrder=Zero-based contiguous  Inputs=8  zeroidx=on  OutDataTypeStr=fixdt(1, 28, 12)  SaturateOnIntegerOverflow=off
  Symbol Demodulator : whdlmod/Symbol Demodulator  ModulationSource=Property  ModulationScheme=BPSK  MaxModulation=256-QAM  ConstOrder=Default  ConstMap=[ 2, 3, 1, 0, 6, 7, 5, 4, 14, 15, 13, 12, 10, 11, 9, 8 ]  DecisionType=Approximate log-likelihood ratio  PhaseOffset=0  OutputType=Vector  NormMethod=Unit average power  MinSymDistance=2  NoiseVariance=off  SimulateUsing=Code generation
  Symbol Demodulator1 : whdlmod/Symbol Demodulator  ModulationSource=Property  ModulationScheme=QPSK  MaxModulation=256-QAM  ConstOrder=Default  ConstMap=[ 2, 3, 1, 0, 6, 7, 5, 4, 14, 15, 13, 12, 10, 11, 9, 8 ]  DecisionType=Approximate log-likelihood ratio  PhaseOffset=-pi/4  OutputType=Vector  NormMethod=Unit average power  MinSymDistance=2  NoiseVariance=off  SimulateUsing=Code generation
  Symbol Demodulator1_term1 : Terminator
  Symbol Demodulator2 : whdlmod/Symbol Demodulator  ModulationSource=Property  ModulationScheme=16-QAM  MaxModulation=256-QAM  ConstOrder=Default  ConstMap=qamFourBits.'  DecisionType=Approximate log-likelihood ratio  PhaseOffset=pi/2  OutputType=Vector  NormMethod=Unit average power  MinSymDistance=2  NoiseVariance=off  SimulateUsing=Code generation
  Symbol Demodulator2_term1 : Terminator
  Symbol Demodulator_term1 : Terminator
  to_12bit_integer : Subsystem
  data_out : Outport  SampleTime=2e-08
  valid_out : Outport  Port=2  SampleTime=2e-08
  wires:
  to_12bit_integer/3(4bit_out) -> Multiport Switch/6
  to_12bit_integer/2(2bit_out) -> Multiport Switch/4
  to_12bit_integer/1(1bit_out) -> Multiport Switch/2, Multiport Switch/3
  Symbol Demodulator2/2 -> Symbol Demodulator2_term1/1
  Symbol Demodulator2/1 -> Delay4/1
  Symbol Demodulator1/2 -> Symbol Demodulator1_term1/1
  Symbol Demodulator1/1 -> Delay3/1
  Symbol Demodulator/2 -> Symbol Demodulator_term1/1
  Symbol Demodulator/1 -> Delay2/1
  Multiport Switch/1 -> Delay/1
  Delay7/1 -> Multiport Switch/1
  Delay5/1 -> Delay1/1
  Delay4/1 -> to_12bit_integer/3(4bit)
  Delay3/1 -> to_12bit_integer/2(2bit)
  Delay2/1 -> to_12bit_integer/1(1bit)
  Delay1/1 -> valid_out/1
  Delay/1 -> data_out/1
  Constant5/1 -> Multiport Switch/9
  Constant4/1 -> Multiport Switch/8
  Constant2/1 -> Multiport Switch/5
  Constant1/1 -> Multiport Switch/7
  bits_per_subcarrier/1 -> Delay7/1
  valid_in/1 -> Symbol Demodulator2/2, Symbol Demodulator1/2, Symbol Demodulator/2, Delay5/1
  data_in/1 -> Symbol Demodulator2/1, Symbol Demodulator1/1, Symbol Demodulator/1

== system gm_HDLRx_vs/full_rx/rx_demodulator_full/rising_edge_detector ==
  In : Inport  OutDataTypeStr=boolean  SampleTime=2e-08
  Delay2 : Delay  DelayLength=1  InitialCondition=0  UseCircularBuffer=on
  Logical Operator1 : Logic  IconShape=distinctive  AllPortsSameDT=off  OutDataTypeStr=boolean
  Logical Operator2 : Logic  Operator=NOT  IconShape=distinctive  AllPortsSameDT=off  OutDataTypeStr=boolean
  Out : Outport  SampleTime=2e-08
  wires:
  Logical Operator2/1 -> Logical Operator1/2
  Logical Operator1/1 -> Out/1
  Delay2/1 -> Logical Operator2/1
  In/1 -> Delay2/1, Logical Operator1/1

== system gm_HDLRx_vs/full_rx/rx_demodulator_full/rising_edge_detector1 ==
  In : Inport  OutDataTypeStr=boolean  SampleTime=2e-08
  Delay2 : Delay  DelayLength=1  InitialCondition=0  UseCircularBuffer=on
  Logical Operator1 : Logic  IconShape=distinctive  AllPortsSameDT=off  OutDataTypeStr=boolean
  Logical Operator2 : Logic  Operator=NOT  IconShape=distinctive  AllPortsSameDT=off  OutDataTypeStr=boolean
  Out : Outport  SampleTime=2e-08
  wires:
  Logical Operator2/1 -> Logical Operator1/2
  Logical Operator1/1 -> Out/1
  Delay2/1 -> Logical Operator2/1
  In/1 -> Delay2/1, Logical Operator1/1

== system gm_HDLRx_vs/full_rx/rx_demodulator_full/valid_to_mux ==
  valid_channel : Inport  OutDataTypeStr=boolean  PortDimensions=1  SampleTime=2e-08
  valid_header : Inport  Port=2  OutDataTypeStr=boolean  PortDimensions=1  SampleTime=2e-08
  valid_payload : Inport  Port=3  OutDataTypeStr=boolean  PortDimensions=1  SampleTime=2e-08
  Bit Concat : hdlsllib/Logic and Bit Operations/Bit Concat  numInputs=2
  Logical Operator : Logic  Operator=OR  IconShape=distinctive  AllPortsSameDT=off  OutDataTypeStr=boolean
  Logical Operator1 : Logic  Operator=OR  IconShape=distinctive  AllPortsSameDT=off  OutDataTypeStr=boolean
  control : Outport  SampleTime=2e-08
  wires:
  Logical Operator1/1 -> Bit Concat/2
  Logical Operator/1 -> Bit Concat/1
  Bit Concat/1 -> control/1
  valid_payload/1 -> Logical Operator/1, Logical Operator1/1
  valid_header/1 -> Logical Operator/2
  valid_channel/1 -> Logical Operator1/2

== system gm_HDLRx_vs/full_rx/rx_demodulator_full/valid_to_mux1 ==
  valid_channel : Inport  OutDataTypeStr=boolean  PortDimensions=1  SampleTime=2e-08
  valid_header : Inport  Port=2  OutDataTypeStr=boolean  PortDimensions=1  SampleTime=2e-08
  valid_payload : Inport  Port=3  OutDataTypeStr=boolean  PortDimensions=1  SampleTime=2e-08
  Bit Concat : hdlsllib/Logic and Bit Operations/Bit Concat  numInputs=2
  Logical Operator : Logic  Operator=OR  IconShape=distinctive  AllPortsSameDT=off  OutDataTypeStr=boolean
  Logical Operator1 : Logic  Operator=OR  IconShape=distinctive  AllPortsSameDT=off  OutDataTypeStr=boolean
  control : Outport  SampleTime=2e-08
  wires:
  Logical Operator1/1 -> Bit Concat/2
  Logical Operator/1 -> Bit Concat/1
  Bit Concat/1 -> control/1
  valid_payload/1 -> Logical Operator/1, Logical Operator1/1
  valid_header/1 -> Logical Operator/2
  valid_channel/1 -> Logical Operator1/2

== system gm_HDLRx_vs/full_rx/rx_payload_full/next_frame_to_ready_rx ==
  note: Given a next frame rising edge, this subsystem will generate a "ready" signal for the duration of "payloadBitsPerFec" clock cycles
  next_frame : Inport  OutDataTypeStr=boolean  PortDimensions=1  SampleTime=1e-08
  HDL Counter : hdlsllib/Sources/HDL Counter  CountType=Count limited  CountInit=0  CountStep=1  CountMax=payloadBitsPerFec-1  CountFromType=Initial value  CountFrom=0  CountResetPort=off  CountLoadPort=off  CountEnbPort=on  CountDirPort=off  CountHitOutputPort=on  CountDataType=Unsigned  CountWordLen=nextpow2(payloadBitsPerFec)  CountFracLen=0  CountSampTime=1
  HDL Counter_term0 : Terminator
  Logical Operator2 : Logic  Operator=NOT  IconShape=distinctive  AllPortsSameDT=off  OutDataTypeStr=boolean
  Logical Operator3 : Logic  Operator=OR  IconShape=distinctive  AllPortsSameDT=off  OutDataTypeStr=boolean
  Unit Delay Enabled Synchronous : hdlsllib/Discrete/Unit Delay Enabled Synchronous  InitialCondition=0.0  SampleTime=-1
  rising_edge_detector : Subsystem
  ready : Outport  SampleTime=1e-08  VectorParamsAs1DForOutWhenUnconnected=off
  wires:
  rising_edge_detector/1(Out) -> Logical Operator3/1
  Unit Delay Enabled Synchronous/1 -> HDL Counter/1, ready/1
  Logical Operator3/1 -> Unit Delay Enabled Synchronous/2
  Logical Operator2/1 -> Unit Delay Enabled Synchronous/1
  HDL Counter/2 -> Logical Operator2/1, Logical Operator3/2
  HDL Counter/1 -> HDL Counter_term0/1
  next_frame/1 -> rising_edge_detector/1(In)

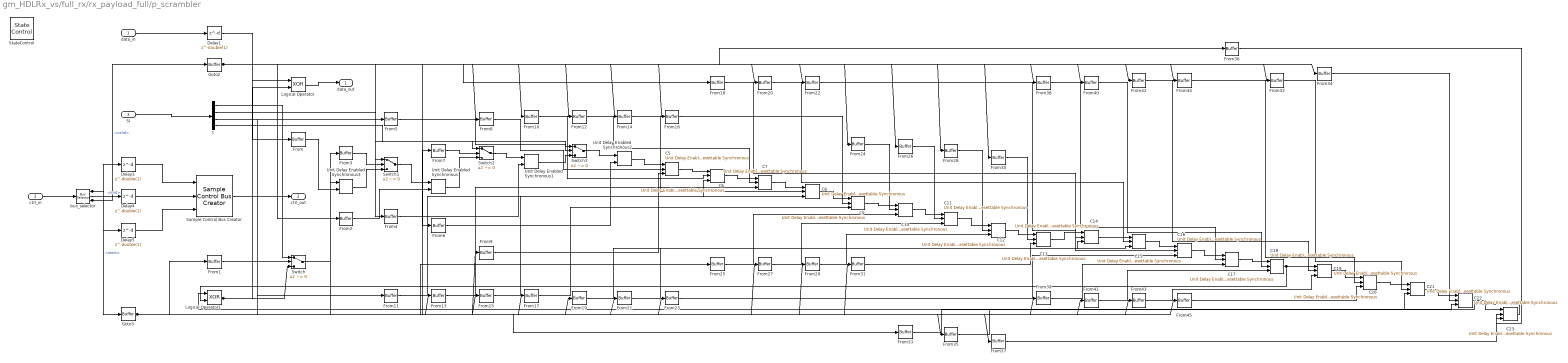
== system gm_HDLRx_vs/full_rx/rx_payload_full/p_scrambler ==
  data_in : Inport  OutDataTypeStr=boolean  SampleTime=1e-08
  ctrl_in : Inport  Port=2  SampleTime=1e-08
  SI : Inport  Port=3  OutDataTypeStr=fixdt(0, 1, 0)  PortDimensions=[4]  SampleTime=1e-08
  C{5..23} (19 alike) : hdlsllib/Discrete/Unit Delay Enabled Resettable Synchronous  InitialCondition=double(1)  SampleTime=-1
  Delay{1,3..5} (4 alike) : Delay  DelayLength=double(1)  InitialCondition=0  SampleTime=1e-08
  From{,1..45} (46 alike) : hdlmdlgenlib/Buffer
  Goto2 : hdlmdlgenlib/Buffer
  Goto3 : hdlmdlgenlib/Buffer
  Logical Operator : Logic  Operator=XOR  AllPortsSameDT=off  OutDataTypeStr=boolean  SampleTime=1e-08
  Logical Operator1 : Logic  Operator=XOR  AllPortsSameDT=off  OutDataTypeStr=boolean  SampleTime=1e-08
  Sample Control Bus Creator : whdlutilities/Sample Control Bus Creator
  StateControl : StateControl  StateControl=Synchronous
  Switch{,1..3} (4 alike) : Switch  Criteria=u2 ~= 0  Threshold=double(0)  OutDataTypeStr=boolean  SampleTime=1e-08  SaturateOnIntegerOverflow=off  InputSameDT=off
  Unit Delay Enabled Synchronous{,1..3} (4 alike) : hdlsllib/Discrete/Unit Delay Enabled Synchronous  InitialCondition=double(1)  SampleTime=-1
  bus_selector : BusSelector  OutputSignals=start,end,valid
  t : Demux
  data_out : Outport  SampleTime=1e-08
  ctrl_out : Outport  Port=2  SampleTime=1e-08
  wires:
  t/4 -> Switch3/1
  t/3 -> Switch2/1
  t/2 -> Switch1/1
  t/1 -> Switch/1
  Goto3/1 -> From1/1, From11/1, From13/1, From15/1, From17/1, From19/1, From21/1, From23/1, From25/1, From27/1, From29/1, From3/1, From31/1, From33/1, From35/1, From37/1, From39/1, From41/1, From43/1, From45/1, From5/1, From7/1, From9/1
  Goto2/1 -> From/1, From10/1, From12/1, From14/1, From16/1, From18/1, From2/1, From20/1, From22/1, From24/1, From26/1, From28/1, From30/1, From32/1, From34/1, From36/1, From38/1, From4/1, From40/1, From42/1, From44/1, From6/1, From8/1
  Unit Delay Enabled Synchronous3/1 -> Switch1/3
  Unit Delay Enabled Synchronous2/1 -> C5/1
  Unit Delay Enabled Synchronous1/1 -> Switch3/3
  Unit Delay Enabled Synchronous/1 -> Switch2/3
  Switch3/1 -> Unit Delay Enabled Synchronous2/1
  Switch2/1 -> Unit Delay Enabled Synchronous1/1
  Switch1/1 -> Unit Delay Enabled Synchronous/1
  Switch/1 -> Unit Delay Enabled Synchronous3/1
  Sample Control Bus Creator/1 -> ctrl_out/1
  Logical Operator1/1 -> Logical Operator/2, Switch/3
  Logical Operator/1 -> data_out/1
  From9/1 -> C5/3
  From8/1 -> C5/2
  From7/1 -> Switch2/2
  From6/1 -> Unit Delay Enabled Synchronous2/2
  From5/1 -> Switch3/2
  From45/1 -> C20/3
  From44/1 -> C20/2
  From43/1 -> C19/3
  From42/1 -> C19/2
  From41/1 -> C18/3
  From40/1 -> C18/2
  From4/1 -> Unit Delay Enabled Synchronous1/2
  From39/1 -> C17/3
  From38/1 -> C17/2
  From37/1 -> C23/3
  From36/1 -> C23/2
  From35/1 -> C22/3
  From34/1 -> C22/2
  From33/1 -> C21/3
  From32/1 -> C21/2
  From31/1 -> C13/3
  From30/1 -> C13/2
  From3/1 -> Switch1/2
  From29/1 -> C12/3
  From28/1 -> C12/2
  From27/1 -> C11/3
  From26/1 -> C11/2
  From25/1 -> C10/3
  From24/1 -> C10/2
  From23/1 -> C16/3
  From22/1 -> C16/2
  From21/1 -> C15/3
  From20/1 -> C15/2
  From2/1 -> Unit Delay Enabled Synchronous/2
  From19/1 -> C14/3
  From18/1 -> C14/2
  From17/1 -> C9/3
  From16/1 -> C9/2
  From15/1 -> C8/3
  From14/1 -> C8/2
  From13/1 -> C7/3
  From12/1 -> C7/2
  From11/1 -> C6/3
  From10/1 -> C6/2
  From1/1 -> Switch/2
  From/1 -> Unit Delay Enabled Synchronous3/2
  Delay5/1 -> Sample Control Bus Creator/3
  Delay4/1 -> Sample Control Bus Creator/2
  Delay3/1 -> Sample Control Bus Creator/1
  Delay1/1 -> Logical Operator/1
  C9/1 -> C10/1
  C8/1 -> C9/1
  C7/1 -> C8/1
  C6/1 -> C7/1
  C5/1 -> C6/1
  C23/1 -> Logical Operator1/1
  C22/1 -> C23/1
  C21/1 -> C22/1
  C20/1 -> C21/1
  C19/1 -> C20/1
  C18/1 -> C19/1, Logical Operator1/2
  C17/1 -> C18/1
  C16/1 -> C17/1
  C15/1 -> C16/1
  C14/1 -> C15/1
  C13/1 -> C14/1
  C12/1 -> C13/1
  C11/1 -> C12/1
  C10/1 -> C11/1
  bus_selector/3 -> Delay5/1, Goto2/1  "<valid>"
  bus_selector/2 -> Delay4/1  "<end>"
  bus_selector/1 -> Delay3/1, Goto3/1  "<start>"
  SI/1 -> t/1
  ctrl_in/1 -> bus_selector/1
  data_in/1 -> Delay1/1

== system gm_HDLRx_vs/full_rx/rx_payload_full/reduced_ldpc_rx ==
  data_in : Inport  OutDataTypeStr=fixdt(1, 16, 12)  PortDimensions=1  SampleTime=1e-08
  ctrl_in : Inport  Port=2
  Hc_12S_B80 : whdledac/LDPC Decoder  ParityCheckMatrix=Hc_12S  BlockSize=80  Algorithm=Min-sum  ScalingFactor=0.75  Termination=Max  SpecifyInputs=Property  NumIterations=ldpcDecoderMaxNumberIterations  MaxNumIterations=8  ParityCheckStatus=off  SimulateUsing=Code generation
  data_out : Outport  SampleTime=1e-08
  ctrl_out : Outport  Port=2
  next_frame : Outport  Port=3  SampleTime=1e-08  VectorParamsAs1DForOutWhenUnconnected=off
  wires:
  Hc_12S_B80/3 -> next_frame/1
  Hc_12S_B80/2 -> ctrl_out/1
  Hc_12S_B80/1 -> data_out/1
  ctrl_in/1 -> Hc_12S_B80/2
  data_in/1 -> Hc_12S_B80/1

== system gm_HDLRx_vs/full_rx/rx_payload_full/remove_tone_mapping ==
  data_in : Inport  OutDataTypeStr=fixdt(1, 16, 12)  SampleTime=1e-08
  valid_in : Inport  Port=2  OutDataTypeStr=boolean  SampleTime=1e-08
  newFrame : Inport  Port=3  OutDataTypeStr=boolean  SampleTime=1e-08
  psdu_size : Inport  Port=4  OutDataTypeStr=fixdt(0, 1, 0)  PortDimensions=[24]  SampleTime=1e-08
  Bits to Word : hdlsllib/Logic and Bit Operations/Bits to Word
  Data Type Conversion : DataTypeConversion  OutDataTypeStr=fixdt(0,1,0)  SaturateOnIntegerOverflow=off  RndMeth=Floor
  Delay : Delay  DelayLength=1  InitialCondition=0  UseCircularBuffer=on
  HDL Counter : hdlsllib/Sources/HDL Counter  CountType=Free running  CountInit=0  CountStep=1  CountMax=25  CountFromType=Initial value  CountFrom=0  CountResetPort=on  CountLoadPort=off  CountEnbPort=on  CountDirPort=off  CountHitOutputPort=off  CountDataType=Unsigned  CountWordLen=32  CountFracLen=0  CountSampTime=1
  Logical Operator : Logic  IconShape=distinctive  AllPortsSameDT=off  OutDataTypeStr=boolean
  Multiply by 2 (for fec_rate 1/2) : hdlsllib/Logic and Bit Operations/Bit Shift  mode=Shift Left Logical  N=1
  Multiply by 8 : hdlsllib/Logic and Bit Operations/Bit Shift  mode=Shift Left Logical  N=3
  Relational Operator : RelationalOperator  Operator=<  OutDataTypeStr=boolean  InputSameDT=off
  valid_to_ctrl : Subsystem
  data_out : Outport  SampleTime=1e-08
  ctrl_out : Outport  Port=2  SampleTime=1e-08
  wires:
  valid_to_ctrl/1(ctrlOut) -> ctrl_out/1
  Relational Operator/1 -> Logical Operator/2
  Multiply by 8/1 -> Multiply by 2 (for fec_rate 1/2)/1
  Multiply by 2 (for fec_rate 1/2)/1 -> Relational Operator/2
  Logical Operator/1 -> valid_to_ctrl/1(validIn)
  HDL Counter/1 -> Relational Operator/1
  Delay/1 -> data_out/1
  Data Type Conversion/1 -> Bits to Word/1
  Bits to Word/1 -> Multiply by 8/1
  psdu_size/1 -> Data Type Conversion/1
  newFrame/1 -> HDL Counter/1
  valid_in/1 -> HDL Counter/2, Logical Operator/1
  data_in/1 -> Delay/1
